simulink model "CraneModel_Final"  (R2022b)
settings: Solver=FixedStepAuto  StartTime=0.0  StopTime=15  FixedStep=0.002  RelTol=1e-3
values from neighbouring files (symbols this model uses):
  fHeightKingActLower = 0.161    [craneParameters.m]
  fHeightKingActUpper = 0.130    (= 0.13)    [craneParameters.m]
  fHeightKingSlew = 0.623    [craneParameters.m]
  fHeightKnuckleActLower = 0.160    (= 0.16)    [craneParameters.m]
  fHeightKnuckleActUpper = 0.182    [craneParameters.m]
  fHeightPlatform = 1.402    [craneParameters.m]
  fHeightPlatformKing = 0.09    [craneParameters.m]
  fHeightSlewTop = 0.711    [craneParameters.m]
  fHeightToSheave1 = 0.060    (= 0.06)    [craneParameters.m]
  fHeightToSheave2 = 0.095    [craneParameters.m]
  fHeightToSheave3 = 0.198    [craneParameters.m]
  fHeightToSheave4 = 1.158    [craneParameters.m]
  fHeightToWinch = 0.0895    [craneParameters.m]
  fLengthKingActLower = 0.154    [craneParameters.m]
  fLengthKingActUpper = 0.600    (= 0.6)    [craneParameters.m]
  fLengthKnuckleActLower = 0.750    (= 0.75)    [craneParameters.m]
  fLengthKnuckleActUpper = 0.027    [craneParameters.m]
  fLengthMainArm = 1.5    [craneParameters.m]
  fLengthPlatform = 1.30    (= 1.3)    [craneParameters.m]
  fLengthToSheave1 = 0.235    [craneParameters.m]
  fLengthToSheave2 = 1.520    (= 1.52)    [craneParameters.m]
  fLengthToSheave3 = 0.168    [craneParameters.m]
  fLengthToSheave4 = 0    [craneParameters.m]
  fLengthToWinch = 0.22    [craneParameters.m]
  fMinLengthActuatorKnuckle = 0.633    [craneParameters.m]
  fMinLengthActuatorMain = 0.691    [craneParameters.m]
  massActuatorBottomMain = 14    [craneParameters.m]
  massActuatorBottomRod = 3    [craneParameters.m]
  massActuatorTopMain = 14    [craneParameters.m]
  massKingBottom = 92.2    [craneParameters.m]
  massKingMountingPlate = 58.2    [craneParameters.m]
  massKingTop = 63.6    [craneParameters.m]
  massKnuckleArm = 8.7    [craneParameters.m]
  massMainArm = 12.5    [craneParameters.m]
  massPayload = 13.5    [craneParameters.m]
  massTestRigBase = 924    [craneParameters.m]
  massTestRigPlatform = 268    [craneParameters.m]
  massWinch = 4.8    [craneParameters.m]
  massWinchDrum = 2.3    [craneParameters.m]
  sheavePitchRadius = sheavePitchDiameter/2    (= 0.034)    [craneParameters.m]
  winchGearRatio = 32    [craneParameters.m]    (also in winchCalculations.m)
undefined symbols (not defined in the file or in its folder): X, Y, Z
libraries: sm_lib x138, nesl_utility x20, vrlib x1, sldrtlib x1
(part 4 of 4)

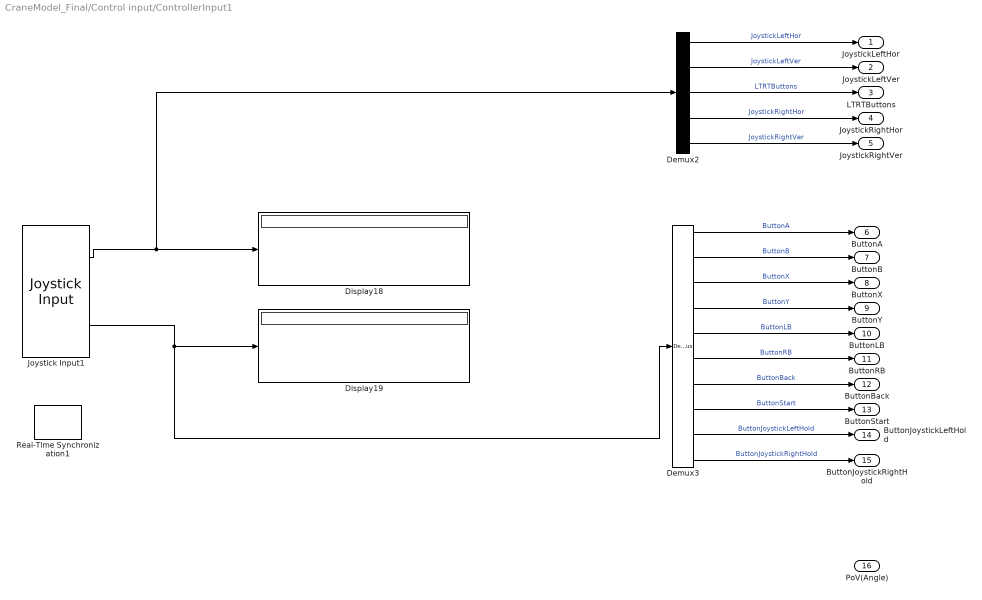
== system CraneModel_Final/Control input/ControllerInput1 ==
  Demux2 : Demux  Outputs=5
  Demux3 : Demux  Outputs=10
  Display18 : Display
  Display19 : Display
  Joystick Input1 : vrlib/Joystick Input  joyid=1  adjustports=on  forcefeed=off
  Real-Time Synchronization1 : sldrtlib/Real-Time Synchronization  SampleTime=0.002  MaxMissedTicks=1000000  ShowMissedTicks=off  YieldWhenWaiting=off
  JoystickLeftHor : Outport
  JoystickLeftVer : Outport  Port=2
  LTRTButtons : Outport  Port=3
  JoystickRightHor : Outport  Port=4
  JoystickRightVer : Outport  Port=5
  ButtonA : Outport  Port=6
  ButtonB : Outport  Port=7
  ButtonX : Outport  Port=8
  ButtonY : Outport  Port=9
  ButtonLB : Outport  Port=10
  ButtonRB : Outport  Port=11
  ButtonBack : Outport  Port=12
  ButtonStart : Outport  Port=13
  ButtonJoystickLeftHold : Outport  Port=14
  ButtonJoystickRightHold : Outport  Port=15
  PoV(Angle) : Outport  Port=16
  wires:
  Joystick Input1/2 -> Display19/1, Demux3/1
  Demux3/1 -> ButtonA/1  "ButtonA"
  Joystick Input1/1 -> Demux2/1, Display18/1
  Demux2/2 -> JoystickLeftVer/1  "JoystickLeftVer"
  Demux2/3 -> LTRTButtons/1  "LTRTButtons"
  Demux3/5 -> ButtonLB/1  "ButtonLB"
  Demux3/3 -> ButtonX/1  "ButtonX"
  Demux2/1 -> JoystickLeftHor/1  "JoystickLeftHor"
  Demux3/10 -> ButtonJoystickRightHold/1  "ButtonJoystickRightHold"
  Demux3/6 -> ButtonRB/1  "ButtonRB"
  Demux2/4 -> JoystickRightHor/1  "JoystickRightHor"
  Demux3/9 -> ButtonJoystickLeftHold/1  "ButtonJoystickLeftHold"
  ? -> PoV(Angle)/1  "PoV(Angle)"
  Demux2/5 -> JoystickRightVer/1  "JoystickRightVer"
  Demux3/7 -> ButtonBack/1  "ButtonBack"
  Demux3/8 -> ButtonStart/1  "ButtonStart"
  Demux3/4 -> ButtonY/1  "ButtonY"
  Demux3/2 -> ButtonB/1  "ButtonB"

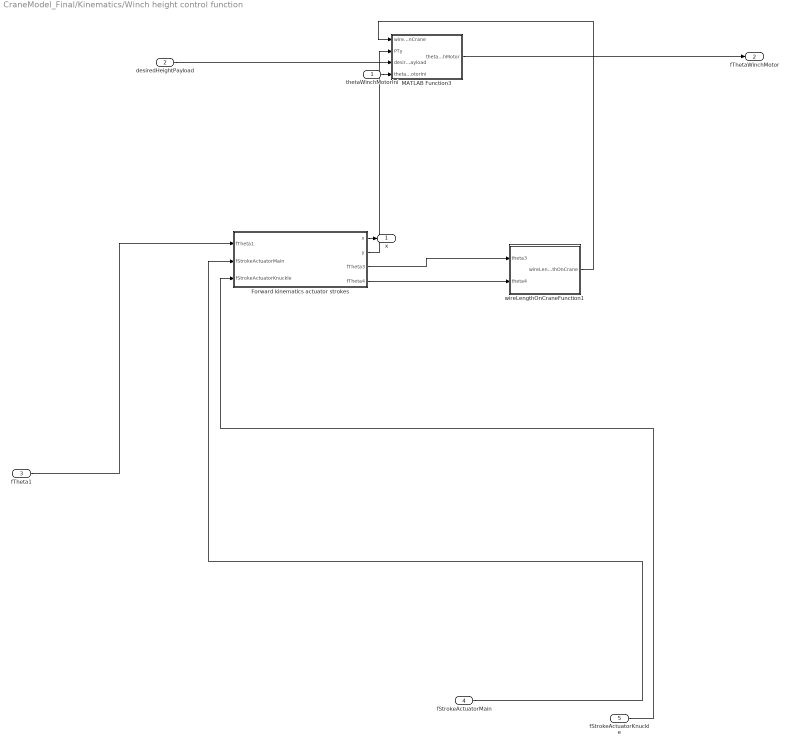
== system CraneModel_Final/Kinematics/Winch height control function ==
  thetaWinchMotorIni : Inport
  desiredHeightPayload : Inport  Port=2
  fTheta1 : Inport  Port=3
  fStrokeActuatorMain : Inport  Port=4
  fStrokeActuatorKnuckle : Inport  Port=5
  Forward kinematics actuator strokes : MATLAB Function  TreatAsAtomicUnit=on
  MATLAB Function3 : MATLAB Function  TreatAsAtomicUnit=on
  wireLengthOnCraneFunction1 : MATLAB Function  TreatAsAtomicUnit=on
  x : Outport
  fThetaWinchMotor : Outport  Port=2
  wires:
  MATLAB Function3/1(thetaWinchMotor) -> fThetaWinchMotor/1
  wireLengthOnCraneFunction1/1(wireLengthOnCrane) -> MATLAB Function3/1(wireLengthOnCrane)
  fStrokeActuatorKnuckle/1 -> Forward kinematics actuator strokes/3(fStrokeActuatorKnuckle)
  Forward kinematics actuator strokes/4(fTheta4) -> wireLengthOnCraneFunction1/2(theta4)
  desiredHeightPayload/1 -> MATLAB Function3/3(desiredHeightPayload)
  fStrokeActuatorMain/1 -> Forward kinematics actuator strokes/2(fStrokeActuatorMain)
  Forward kinematics actuator strokes/2(y) -> MATLAB Function3/2(PTy)
  Forward kinematics actuator strokes/3(fTheta3) -> wireLengthOnCraneFunction1/1(theta3)
  Forward kinematics actuator strokes/1(x) -> x/1
  thetaWinchMotorIni/1 -> MATLAB Function3/4(thetaWinchMotorIni)
  fTheta1/1 -> Forward kinematics actuator strokes/1(fTheta1)

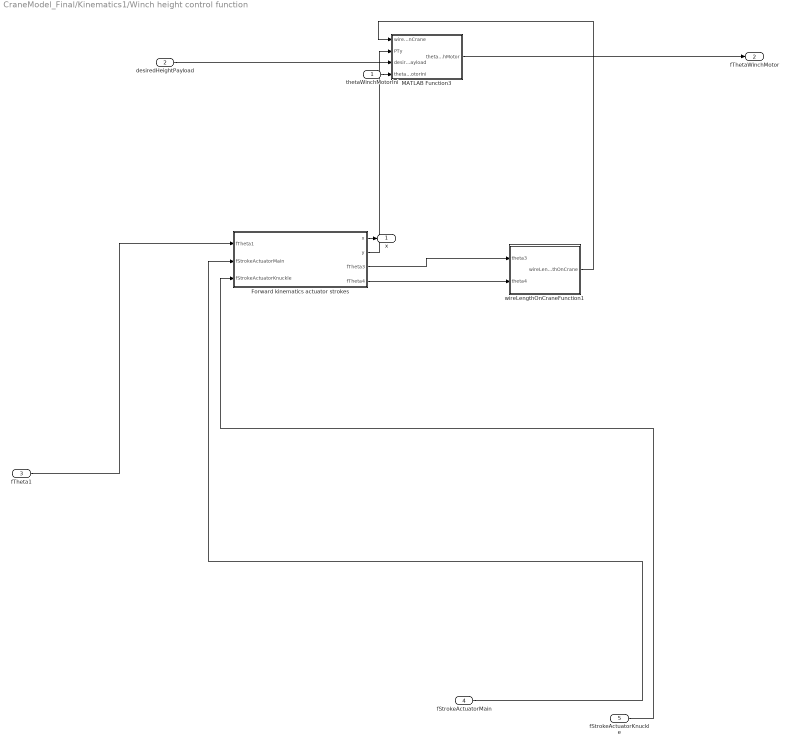
== system CraneModel_Final/Kinematics1/Winch height control function ==
  thetaWinchMotorIni : Inport
  desiredHeightPayload : Inport  Port=2
  fTheta1 : Inport  Port=3
  fStrokeActuatorMain : Inport  Port=4
  fStrokeActuatorKnuckle : Inport  Port=5
  Forward kinematics actuator strokes : MATLAB Function  TreatAsAtomicUnit=on
  MATLAB Function3 : MATLAB Function  TreatAsAtomicUnit=on
  wireLengthOnCraneFunction1 : MATLAB Function  TreatAsAtomicUnit=on
  x : Outport
  fThetaWinchMotor : Outport  Port=2
  wires:
  MATLAB Function3/1(thetaWinchMotor) -> fThetaWinchMotor/1
  wireLengthOnCraneFunction1/1(wireLengthOnCrane) -> MATLAB Function3/1(wireLengthOnCrane)
  fStrokeActuatorKnuckle/1 -> Forward kinematics actuator strokes/3(fStrokeActuatorKnuckle)
  Forward kinematics actuator strokes/4(fTheta4) -> wireLengthOnCraneFunction1/2(theta4)
  desiredHeightPayload/1 -> MATLAB Function3/3(desiredHeightPayload)
  fStrokeActuatorMain/1 -> Forward kinematics actuator strokes/2(fStrokeActuatorMain)
  Forward kinematics actuator strokes/2(y) -> MATLAB Function3/2(PTy)
  Forward kinematics actuator strokes/3(fTheta3) -> wireLengthOnCraneFunction1/1(theta3)
  Forward kinematics actuator strokes/1(x) -> x/1
  thetaWinchMotorIni/1 -> MATLAB Function3/4(thetaWinchMotorIni)
  fTheta1/1 -> Forward kinematics actuator strokes/1(fTheta1)

== matlab function CraneModel_Final/Kinematics/Winch height control function/Forward kinematics actuator strokes ==
  data: fTheta1 input; x output; y output; fStrokeActuatorMain input; fStrokeActuatorKnuckle input; fTheta3 output; fTheta4 output
function [x, y, fTheta3, fTheta4] = fcn(fTheta1, fStrokeActuatorMain, fStrokeActuatorKnuckle)

 %Platform constants
fHeightPlatform = 1.402;
fHeightPlatformKing = 0.09;
fLengthPlatform = 1.30;

%Crane and platform dimensions
%Crane constant parameters

fHeightKingSlew             = 0.623;
fHeightSlewTop              = 0.711;
fLengthMainArm			    = 1.5;
fLengthKnuckleArm		    = 1.158;

fLengthAMain				= 0.614;
fLengthBMain				= 0.571;
fMinLengthActuatorMain		= 0.691;
fMaxStrokeActuatorMain		= 0.320;

fOffsetAngleDegMainAct		= 62.1;
fOffsetAngleRadMainAct		= deg2rad(fOffsetAngleDegMainAct);

fLengthAKnuckle				= 0.767;
fLengthBKnuckle				= 0.184;
fMinLengthActuatorKnuckle	= 0.633;
fMaxStrokeActuatorKnuckle	= 0.260;

fOffsetAngleDegKnuckleAct	= 86.3;
fOffsetAngleRadKnuckleAct	= deg2rad(fOffsetAngleDegKnuckleAct);

%Calculating angles for main arm
fLengthActuatorMain = fStrokeActuatorMain + fMinLengthActuatorMain;

fAngleMainArmAct = acos((fLengthBMain^2 + fLengthAMain^2 - fLengthActuatorMain^2) / (2 * fLengthBMain * fLengthAMain));

fTheta3 = fAngleMainArmAct - fOffsetAngleRadMainAct;

%Calculating angles for knuckle arm
fLengthActuatorKnuckle = fStrokeActuatorKnuckle + fMinLengthActuatorKnuckle;

fAngleKnuckleArmAct = acos((fLengthBKnuckle^2 + fLengthAKnuckle^2 - fLengthActuatorKnuckle^2) / (2 * fLengthBKnuckle * fLengthAKnuckle));

fTheta4 = fAngleKnuckleArmAct - fOffsetAngleRadKnuckleAct;


	
% 
% fAngleMainArmAct			= fTheta3deg + fOffsetAngleDegMainAct;
% fAngleKnuckleArmAct         = fTheta4deg + fOffsetAngleDegKnuckleAct;
% 
% fLengthActuatorMain         = sqrt(fLengthAMain^2 + fLengthBMain^2 -(2*fLengthAMain*fLengthBMain*cosd(fAngleMainArmAct)));
% fStrokeActuatorMain         = fLengthActuatorMain - fMinLengthActuatorMain;
% if fStrokeActuatorMain < 0
%     fStrokeActuatorMain = 0;
% elseif fStrokeActuatorMain > fMaxStrokeActuatorMain
%     fMaxStrokeActuatorMain = fMaxStrokeActuatorMain;
% end
% 
% fLengthActuatorKnuckle         = sqrt(fLengthAKnuckle^2 + fLengthBKnuckle^2 -(2*fLengthAKnuckle*fLengthBKnuckle*cosd(fAngleKnuckleArmAct)));
% fStrokeActuatorKnuckle         = fLengthActuatorKnuckle - fMinLengthActuatorKnuckle;
% 
% if fStrokeActuatorKnuckle < 0
%     fStrokeActuatorKnuckle = 0;
% elseif fStrokeActuatorKnuckle > fMaxStrokeActuatorKnuckle
%     fMaxStrokeActuatorKnuckle = fMaxStrokeActuatorKnuckle;
% end



fHeightMain                 = fHeightPlatformKing + fHeightKingSlew + fHeightSlewTop;

% x = fLengthPlatform*cos(fTheta1) + fHeightMain*cos(fTheta1 + pi/2) + fLengthMainArm*cos(fTheta1 + fTheta3) + fLengthKnuckleArm * cos (fTheta1 + fTheta3 + fTheta4 - pi/2);
% y = fHeightPlatform + fLengthPlatform*sin(fTheta1) + fHeightMain * sin(fTheta1 + pi/2) + fLengthMainArm *sin(fTheta1 + fTheta3) + fLengthKnuckleArm*sin(fTheta1 + fTheta3 + fTheta4 - pi/2);

x = fLengthPlatform*cos(fTheta1) + fHeightMain*cos(fTheta1 + pi/2) + fLengthMainArm*cos(fTheta1 + fTheta3) + fLengthKnuckleArm * cos (fTheta1 + fTheta3 + fTheta4 - pi/2);
y = fHeightPlatform + fLengthPlatform*sin(fTheta1) + fHeightMain * sin(fTheta1 + pi/2) + fLengthMainArm *sin(fTheta1 + fTheta3) + fLengthKnuckleArm*sin(fTheta1 + fTheta3 + fTheta4 - pi/2);

== matlab function CraneModel_Final/Kinematics/WinchHeightControlFunction ==
  data: fTheta1 input; PTx output; PTy output; fStrokeActuatorMain input; fStrokeActuatorKnuckle input; fTheta3 output; fTheta4 output; thetaWinchMotorIni input; desiredHeightPayload input; thetaWinchMotor output
function [PTx, PTy, fTheta3, fTheta4, thetaWinchMotor] = fcn(fTheta1, fStrokeActuatorMain, fStrokeActuatorKnuckle, thetaWinchMotorIni, desiredHeightPayload)

 %Platform constants
fHeightPlatform = 1.402;
fHeightPlatformKing = 0.09;
fLengthPlatform = 1.30;

%Crane and platform dimensions
%Crane constant parameters

fHeightKingSlew             = 0.623;
fHeightSlewTop              = 0.711;
fLengthMainArm			    = 1.5;
fLengthKnuckleArm		    = 1.158;

fLengthAMain				= 0.614;
fLengthBMain				= 0.571;
fMinLengthActuatorMain		= 0.691;
fMaxStrokeActuatorMain		= 0.320;

fOffsetAngleDegMainAct		= 62.1;
fOffsetAngleRadMainAct		= deg2rad(fOffsetAngleDegMainAct);

fLengthAKnuckle				= 0.767;
fLengthBKnuckle				= 0.184;
fMinLengthActuatorKnuckle	= 0.633;
fMaxStrokeActuatorKnuckle	= 0.260;

fOffsetAngleDegKnuckleAct	= 86.3;
fOffsetAngleRadKnuckleAct	= deg2rad(fOffsetAngleDegKnuckleAct);

lengthOrigoToWinch = 0.2199;
heightOrigoToWinch = 0.0895;
lengthOrigoToSheave1 = 0.2348;
heightOrigoToSheave1 = 0.060;
lengthOrigoToSheave2 = 1.520;
heigthOrigoToSheave2 = 0.095;
lengthMainArmToSheave3 = 0.2591;
lengthMainArmToSheave4 = 1.158;
offsetAngleSheave3deg = 49.7;
offsetAngleSheave3rad = deg2rad(offsetAngleSheave3deg);
offsetAngleSheave4deg = 90;
offsetAngleSheave4rad = deg2rad(offsetAngleSheave4deg);

lengthMainArm = 1.500;
pitchRadiusWinch = 0.0716;
pitchRadiusSheave = 0.034;

%Calculating angles for main arm
fLengthActuatorMain = fStrokeActuatorMain + fMinLengthActuatorMain;

fAngleMainArmAct = acos((fLengthBMain^2 + fLengthAMain^2 - fLengthActuatorMain^2) / (2 * fLengthBMain * fLengthAMain));

fTheta3 = fAngleMainArmAct - fOffsetAngleRadMainAct;

%Calculating angles for knuckle arm
fLengthActuatorKnuckle = fStrokeActuatorKnuckle + fMinLengthActuatorKnuckle;

fAngleKnuckleArmAct = acos((fLengthBKnuckle^2 + fLengthAKnuckle^2 - fLengthActuatorKnuckle^2) / (2 * fLengthBKnuckle * fLengthAKnuckle));

fTheta4 = fAngleKnuckleArmAct - fOffsetAngleRadKnuckleAct;


fHeightMain = fHeightPlatformKing + fHeightKingSlew + fHeightSlewTop;

PTx = fLengthPlatform*cos(fTheta1) + fHeightMain*cos(fTheta1 + pi/2) + fLengthMainArm*cos(fTheta1 + fTheta3) + fLengthKnuckleArm * cos (fTheta1 + fTheta3 + fTheta4 - pi/2);
PTy = fHeightPlatform + fLengthPlatform*sin(fTheta1) + fHeightMain * sin(fTheta1 + pi/2) + fLengthMainArm *sin(fTheta1 + fTheta3) + fLengthKnuckleArm*sin(fTheta1 + fTheta3 + fTheta4 - pi/2);


Pwx = -lengthOrigoToWinch;
Pwy = -heightOrigoToWinch;
Ps1x = lengthOrigoToSheave1 * cos(fTheta3) - heightOrigoToSheave1 * sin(fTheta3);
Ps1y = lengthOrigoToSheave1 * sin(fTheta3) + heightOrigoToSheave1 * cos(fTheta3);
Ps2x = lengthOrigoToSheave2 * cos(fTheta3) - heigthOrigoToSheave2 * sin(fTheta3);
Ps2y = lengthOrigoToSheave2 * sin(fTheta3) + heigthOrigoToSheave2 * cos(fTheta3);
Ps3x = lengthMainArm * cos(fTheta3) + lengthMainArmToSheave3 * cos(fTheta3 + fTheta4 - offsetAngleSheave3rad);
Ps3y = lengthMainArm * sin(fTheta3) + lengthMainArmToSheave3 * sin(fTheta3 + fTheta4 - offsetAngleSheave3rad); 
Ps4x = lengthMainArm * cos(fTheta3) + lengthMainArmToSheave4 * cos(fTheta3 + fTheta4 - offsetAngleSheave4rad);
Ps4y = lengthMainArm * sin(fTheta3) + lengthMainArmToSheave4 * sin(fTheta3 + fTheta4 - offsetAngleSheave4rad);

%  function distance = distanceTwoPoints(P1x, P1y, P2x, P2y)
%        distance = sqrt((P2x - P1x)^2 + (P2y - P1y)^2);
%    end

distanceWinchSheave1 =  sqrt((Ps1x - Pwx)^2 + (Ps1y - Pwy)^2); %distanceTwoPoints(Pwx, Pwy, Ps1x, Ps1y);
distanceSheave1Sheave2 = sqrt((Ps2x - Ps1x)^2 + (Ps2y - Ps1y)^2); %distanceTwoPoints(Ps2x, Ps2y, Ps1x, Ps1y);
distanceSheave2Sheave3 = sqrt((Ps3x - Ps2x)^2 + (Ps3y - Ps2y)^2); %distanceTwoPoints(Ps2x, Ps2y, Ps3x, Ps3y);
distanceSheave3Sheave4 = sqrt((Ps4x - Ps3x)^2 + (Ps4y - Ps3y)^2); %distanceTwoPoints(Ps4x, Ps4y, Ps3x, Ps3y);

% function tangentLength = tangentLengthFunction(distance, radius1, radius2)
%         tangentLength = sqrt(distance^2 -(radius1 -radius2)^2);
%     end

tangentLengthWinchSheave1 = sqrt(distanceWinchSheave1^2 -(pitchRadiusWinch -pitchRadiusSheave)^2); %tangentLengthFunction(distanceWinchSheave1, pitchRadiusWinch, pitchRadiusSheave);
tangentLengthSheave1Sheave2 = sqrt(distanceSheave1Sheave2^2 -(pitchRadiusSheave -pitchRadiusSheave)^2); %tangentLengthFunction(distanceSheave1Sheave2, pitchRadiusSheave, pitchRadiusSheave);
tangentLengthSheave2Sheave3 = sqrt(distanceSheave2Sheave3^2 -(pitchRadiusSheave -pitchRadiusSheave)^2); %tangentLengthFunction(distanceSheave2Sheave3, pitchRadiusSheave, pitchRadiusSheave);
tangentLengthSheave3Sheave4 = sqrt(distanceSheave3Sheave4^2 -(pitchRadiusSheave -pitchRadiusSheave)^2); %tangentLengthFunction(distanceSheave3Sheave4, pitchRadiusSheave, pitchRadiusSheave);

offsetAngleDeg = 113.6 + 9.9;
offsetAngleRad = deg2rad(offsetAngleDeg);

wrapAngle = offsetAngleRad - fTheta3 - fTheta4;
wrapLength = wrapAngle * pitchRadiusSheave;

wireLengthOnCrane = tangentLengthWinchSheave1 + tangentLengthSheave1Sheave2 + tangentLengthSheave2Sheave3 + tangentLengthSheave3Sheave4 + wrapLength;

lengthWinchWireIni = 3;
pitchRadiusWinch = 0.0716;
pitchRadiusSheave = 0.034;
gearRatioWinch = 32;

lengthWinchWire = PTy - desiredHeightPayload;
thetaWinch = (lengthWinchWire - lengthWinchWireIni) / pitchRadiusWinch;
thetaWinchMotor = thetaWinch*gearRatioWinch + thetaWinchMotorIni;

%     function distance = distanceTwoPoints(P1x, P1y, P2x, P2y)
%         distance = sqrt((P2x - P1x)^2 + (P2y - P1y)^2);
%     end
% 
%     function tangentLength = tangentLengthFunction(distance, radius1, radius2)
%         tangentLength = sqrt(distance^2 -(radius1 -radius2)^2);
%     end
end

== matlab function CraneModel_Final/Kinematics1/Inverse kinematics function ==
  data: fPtXd input; fPtYd input; fStrokeActuatorMain output; fStrokeActuatorKnuckle output; fTheta1 input; fTheta3 output; fTheta4 output
function [fStrokeActuatorMain, fStrokeActuatorKnuckle, fTheta3, fTheta4] = fcn(fPtXd, fPtYd, fTheta1)
    
    %Platform constants
    h0 = 1.402;
    l0 = 1.3;
    
    %Crane constants
    h1 = 1.334 + 0.09;
    lm = 1.5;
    lk = 1.158;

    %Calculate position of a2 as function of Theta1
    a2x = l0*cos(fTheta1) + h1*cos(fTheta1 + pi/2);
    a2y = h0 + l0*sin(fTheta1) + h1*sin(fTheta1 + pi/2);

    h = sqrt((fPtXd - a2x)^2 + (fPtYd - a2y)^2);
    phi = atan((fPtYd - a2y) / (fPtXd - a2x));
    
    %Calculate ThetaA and ThetaB
    ThetaA = acos ((lm^2 + h^2 - lk^2) / (2*lm*h));
    ThetaB = acos ((lk^2 + lm^2 - h^2) / (2*lm*lk));

    fTheta3 = ThetaA + phi - fTheta1;
    fTheta4 = ThetaB - pi/2;

    fTheta3deg = rad2deg(fTheta3);
    fTheta4deg = rad2deg(fTheta4);

	%Crane constant parameters
	fLengthP2PMainArm			= lm;
	fLengthP2PKnuckleArm		= lk;
	
	fLengthAMain				= 0.614;
	fLengthBMain				= 0.571;
	fMinLengthActuatorMain		= 0.691;
	fMaxStrokeActuatorMain		= 0.320;
	
    fOffsetAngleDegMainAct		= 62.1;
	
	fLengthAKnuckle				= 0.767;
	fLengthBKnuckle				= 0.184;
	fMinLengthActuatorKnuckle	= 0.633;
	fMaxStrokeActuatorKnuckle	= 0.260;
	
    fOffsetAngleDegKnuckleAct	= 86.3;
	

fAngleMainArmAct			= fTheta3deg + fOffsetAngleDegMainAct;
fAngleKnuckleArmAct         = fTheta4deg + fOffsetAngleDegKnuckleAct;

fLengthActuatorMain         = sqrt(fLengthAMain^2 + fLengthBMain^2 -(2*fLengthAMain*fLengthBMain*cosd(fAngleMainArmAct)));
fStrokeActuatorMain         = fLengthActuatorMain - fMinLengthActuatorMain;

if fStrokeActuatorMain < 0
    fStrokeActuatorMain = 0;
elseif fStrokeActuatorMain > fMaxStrokeActuatorMain
    fMaxStrokeActuatorMain = fMaxStrokeActuatorMain;
end

fLengthActuatorKnuckle         = sqrt(fLengthAKnuckle^2 + fLengthBKnuckle^2 -(2*fLengthAKnuckle*fLengthBKnuckle*cosd(fAngleKnuckleArmAct)));
fStrokeActuatorKnuckle         = fLengthActuatorKnuckle - fMinLengthActuatorKnuckle;

if fStrokeActuatorKnuckle < 0
    fStrokeActuatorKnuckle = 0;
elseif fStrokeActuatorKnuckle > fMaxStrokeActuatorKnuckle
    fMaxStrokeActuatorKnuckle = fMaxStrokeActuatorKnuckle;
end

== matlab function CraneModel_Final/Kinematics1/Winch height control function/Forward kinematics actuator strokes ==
  data: fTheta1 input; x output; y output; fStrokeActuatorMain input; fStrokeActuatorKnuckle input; fTheta3 output; fTheta4 output
function [x, y, fTheta3, fTheta4] = fcn(fTheta1, fStrokeActuatorMain, fStrokeActuatorKnuckle)

 %Platform constants
fHeightPlatform = 1.402;
fHeightPlatformKing = 0.09;
fLengthPlatform = 1.30;

%Crane and platform dimensions
%Crane constant parameters

fHeightKingSlew             = 0.623;
fHeightSlewTop              = 0.711;
fLengthMainArm			    = 1.5;
fLengthKnuckleArm		    = 1.158;

fLengthAMain				= 0.614;
fLengthBMain				= 0.571;
fMinLengthActuatorMain		= 0.691;
fMaxStrokeActuatorMain		= 0.320;

fOffsetAngleDegMainAct		= 62.1;
fOffsetAngleRadMainAct		= deg2rad(fOffsetAngleDegMainAct);

fLengthAKnuckle				= 0.767;
fLengthBKnuckle				= 0.184;
fMinLengthActuatorKnuckle	= 0.633;
fMaxStrokeActuatorKnuckle	= 0.260;

fOffsetAngleDegKnuckleAct	= 86.3;
fOffsetAngleRadKnuckleAct	= deg2rad(fOffsetAngleDegKnuckleAct);

%Calculating angles for main arm
fLengthActuatorMain = fStrokeActuatorMain + fMinLengthActuatorMain;

fAngleMainArmAct = acos((fLengthBMain^2 + fLengthAMain^2 - fLengthActuatorMain^2) / (2 * fLengthBMain * fLengthAMain));

fTheta3 = fAngleMainArmAct - fOffsetAngleRadMainAct;

%Calculating angles for knuckle arm
fLengthActuatorKnuckle = fStrokeActuatorKnuckle + fMinLengthActuatorKnuckle;

fAngleKnuckleArmAct = acos((fLengthBKnuckle^2 + fLengthAKnuckle^2 - fLengthActuatorKnuckle^2) / (2 * fLengthBKnuckle * fLengthAKnuckle));

fTheta4 = fAngleKnuckleArmAct - fOffsetAngleRadKnuckleAct;


	
% 
% fAngleMainArmAct			= fTheta3deg + fOffsetAngleDegMainAct;
% fAngleKnuckleArmAct         = fTheta4deg + fOffsetAngleDegKnuckleAct;
% 
% fLengthActuatorMain         = sqrt(fLengthAMain^2 + fLengthBMain^2 -(2*fLengthAMain*fLengthBMain*cosd(fAngleMainArmAct)));
% fStrokeActuatorMain         = fLengthActuatorMain - fMinLengthActuatorMain;
% if fStrokeActuatorMain < 0
%     fStrokeActuatorMain = 0;
% elseif fStrokeActuatorMain > fMaxStrokeActuatorMain
%     fMaxStrokeActuatorMain = fMaxStrokeActuatorMain;
% end
% 
% fLengthActuatorKnuckle         = sqrt(fLengthAKnuckle^2 + fLengthBKnuckle^2 -(2*fLengthAKnuckle*fLengthBKnuckle*cosd(fAngleKnuckleArmAct)));
% fStrokeActuatorKnuckle         = fLengthActuatorKnuckle - fMinLengthActuatorKnuckle;
% 
% if fStrokeActuatorKnuckle < 0
%     fStrokeActuatorKnuckle = 0;
% elseif fStrokeActuatorKnuckle > fMaxStrokeActuatorKnuckle
%     fMaxStrokeActuatorKnuckle = fMaxStrokeActuatorKnuckle;
% end



fHeightMain                 = fHeightPlatformKing + fHeightKingSlew + fHeightSlewTop;

% x = fLengthPlatform*cos(fTheta1) + fHeightMain*cos(fTheta1 + pi/2) + fLengthMainArm*cos(fTheta1 + fTheta3) + fLengthKnuckleArm * cos (fTheta1 + fTheta3 + fTheta4 - pi/2);
% y = fHeightPlatform + fLengthPlatform*sin(fTheta1) + fHeightMain * sin(fTheta1 + pi/2) + fLengthMainArm *sin(fTheta1 + fTheta3) + fLengthKnuckleArm*sin(fTheta1 + fTheta3 + fTheta4 - pi/2);

x = fLengthPlatform*cos(fTheta1) + fHeightMain*cos(fTheta1 + pi/2) + fLengthMainArm*cos(fTheta1 + fTheta3) + fLengthKnuckleArm * cos (fTheta1 + fTheta3 + fTheta4 - pi/2);
y = fHeightPlatform + fLengthPlatform*sin(fTheta1) + fHeightMain * sin(fTheta1 + pi/2) + fLengthMainArm *sin(fTheta1 + fTheta3) + fLengthKnuckleArm*sin(fTheta1 + fTheta3 + fTheta4 - pi/2);

== matlab function CraneModel_Final/Kinematics1/Winch height control function/MATLAB Function3 ==
  data: wireLengthOnCrane input; PTy input; thetaWinchMotor output; desiredHeightPayload input; thetaWinchMotorIni input
function thetaWinchMotor = fcn(wireLengthOnCrane, PTy, desiredHeightPayload, thetaWinchMotorIni)

lengthWinchWireIni = 3;
pitchRadiusWinch = 0.0716;
pitchRadiusSheave = 0.034;
gearRatioWinch = 32;

lengthWinchWire = PTy - desiredHeightPayload;
thetaWinch = (lengthWinchWire - lengthWinchWireIni) / pitchRadiusWinch;
thetaWinchMotor = thetaWinch*gearRatioWinch + thetaWinchMotorIni;

== matlab function CraneModel_Final/Kinematics1/Winch height control function/wireLengthOnCraneFunction1 ==
  data: theta3 input; wireLengthOnCrane output; theta4 input
function wireLengthOnCrane = fcn(theta3, theta4)

lengthOrigoToWinch = 0.2199;
heightOrigoToWinch = 0.0895;
lengthOrigoToSheave1 = 0.2348;
heightOrigoToSheave1 = 0.060;
lengthOrigoToSheave2 = 1.520;
heigthOrigoToSheave2 = 0.095;
lengthMainArmToSheave3 = 0.2591;
lengthMainArmToSheave4 = 1.158;
offsetAngleSheave3deg = 49.7;
offsetAngleSheave3rad = deg2rad(offsetAngleSheave3deg);
offsetAngleSheave4deg = 90;
offsetAngleSheave4rad = deg2rad(offsetAngleSheave4deg);

lengthMainArm = 1.500;
pitchRadiusWinch = 0.0716;
pitchRadiusSheave = 0.034;

Pwx = -lengthOrigoToWinch;
Pwy = -heightOrigoToWinch;
Ps1x = lengthOrigoToSheave1 * cos(theta3) - heightOrigoToSheave1 * sin(theta3);
Ps1y = lengthOrigoToSheave1 * sin(theta3) + heightOrigoToSheave1 * cos(theta3);
Ps2x = lengthOrigoToSheave2 * cos(theta3) - heigthOrigoToSheave2 * sin(theta3);
Ps2y = lengthOrigoToSheave2 * sin(theta3) + heigthOrigoToSheave2 * cos(theta3);
Ps3x = lengthMainArm * cos(theta3) + lengthMainArmToSheave3 * cos(theta3 + theta4 - offsetAngleSheave3rad);
Ps3y = lengthMainArm * sin(theta3) + lengthMainArmToSheave3 * sin(theta3 + theta4 - offsetAngleSheave3rad); 
Ps4x = lengthMainArm * cos(theta3) + lengthMainArmToSheave4 * cos(theta3 + theta4 - offsetAngleSheave4rad);
Ps4y = lengthMainArm * sin(theta3) + lengthMainArmToSheave4 * sin(theta3 + theta4 - offsetAngleSheave4rad);

distanceWinchSheave1 = distanceTwoPoints(Pwx, Pwy, Ps1x, Ps1y);
distanceSheave1Sheave2 = distanceTwoPoints(Ps2x, Ps2y, Ps1x, Ps1y);
distanceSheave2Sheave3 = distanceTwoPoints(Ps2x, Ps2y, Ps3x, Ps3y);
distanceSheave3Sheave4 = distanceTwoPoints(Ps4x, Ps4y, Ps3x, Ps3y);

tangentLengthWinchSheave1 = tangentLengthFunction(distanceWinchSheave1, pitchRadiusWinch, pitchRadiusSheave);
tangentLengthSheave1Sheave2 = tangentLengthFunction(distanceSheave1Sheave2, pitchRadiusSheave, pitchRadiusSheave);
tangentLengthSheave2Sheave3 = tangentLengthFunction(distanceSheave2Sheave3, pitchRadiusSheave, pitchRadiusSheave);
tangentLengthSheave3Sheave4 = tangentLengthFunction(distanceSheave3Sheave4, pitchRadiusSheave, pitchRadiusSheave);

offsetAngleDeg = 113.6 + 9.9;
offsetAngleRad = deg2rad(offsetAngleDeg);

wrapAngle = offsetAngleRad - theta3 - theta4;
wrapLength = wrapAngle * pitchRadiusSheave;

wireLengthOnCrane = tangentLengthWinchSheave1 + tangentLengthSheave1Sheave2 + tangentLengthSheave2Sheave3 + tangentLengthSheave3Sheave4 + wrapLength;

    function distance = distanceTwoPoints(P1x, P1y, P2x, P2y)
        distance = sqrt((P2x - P1x)^2 + (P2y - P1y)^2);
    end

    function tangentLength = tangentLengthFunction(distance, radius1, radius2)
        tangentLength = sqrt(distance^2 -(radius1 -radius2)^2);
    end
end

== matlab function CraneModel_Final/Kinematics1/WinchHeightControlFunction ==
  data: fTheta1 input; PTx output; PTy output; fStrokeActuatorMain input; fStrokeActuatorKnuckle input; fTheta3 output; fTheta4 output; thetaWinchMotorIni input; desiredHeightPayload input; thetaWinchMotor output
function [PTx, PTy, fTheta3, fTheta4, thetaWinchMotor] = fcn(fTheta1, fStrokeActuatorMain, fStrokeActuatorKnuckle, thetaWinchMotorIni, desiredHeightPayload)

 %Platform constants
fHeightPlatform = 1.402;
fHeightPlatformKing = 0.09;
fLengthPlatform = 1.30;

%Crane and platform dimensions
%Crane constant parameters

fHeightKingSlew             = 0.623;
fHeightSlewTop              = 0.711;
fLengthMainArm			    = 1.5;
fLengthKnuckleArm		    = 1.158;

fLengthAMain				= 0.614;
fLengthBMain				= 0.571;
fMinLengthActuatorMain		= 0.691;
fMaxStrokeActuatorMain		= 0.320;

fOffsetAngleDegMainAct		= 62.1;
fOffsetAngleRadMainAct		= deg2rad(fOffsetAngleDegMainAct);

fLengthAKnuckle				= 0.767;
fLengthBKnuckle				= 0.184;
fMinLengthActuatorKnuckle	= 0.633;
fMaxStrokeActuatorKnuckle	= 0.260;

fOffsetAngleDegKnuckleAct	= 86.3;
fOffsetAngleRadKnuckleAct	= deg2rad(fOffsetAngleDegKnuckleAct);

lengthOrigoToWinch = 0.2199;
heightOrigoToWinch = 0.0895;
lengthOrigoToSheave1 = 0.2348;
heightOrigoToSheave1 = 0.060;
lengthOrigoToSheave2 = 1.520;
heigthOrigoToSheave2 = 0.095;
lengthMainArmToSheave3 = 0.2591;
lengthMainArmToSheave4 = 1.158;
offsetAngleSheave3deg = 49.7;
offsetAngleSheave3rad = deg2rad(offsetAngleSheave3deg);
offsetAngleSheave4deg = 90;
offsetAngleSheave4rad = deg2rad(offsetAngleSheave4deg);

lengthMainArm = 1.500;
pitchRadiusWinch = 0.0716;
pitchRadiusSheave = 0.034;

%Calculating angles for main arm
fLengthActuatorMain = fStrokeActuatorMain + fMinLengthActuatorMain;

fAngleMainArmAct = acos((fLengthBMain^2 + fLengthAMain^2 - fLengthActuatorMain^2) / (2 * fLengthBMain * fLengthAMain));

fTheta3 = fAngleMainArmAct - fOffsetAngleRadMainAct;

%Calculating angles for knuckle arm
fLengthActuatorKnuckle = fStrokeActuatorKnuckle + fMinLengthActuatorKnuckle;

fAngleKnuckleArmAct = acos((fLengthBKnuckle^2 + fLengthAKnuckle^2 - fLengthActuatorKnuckle^2) / (2 * fLengthBKnuckle * fLengthAKnuckle));

fTheta4 = fAngleKnuckleArmAct - fOffsetAngleRadKnuckleAct;


fHeightMain = fHeightPlatformKing + fHeightKingSlew + fHeightSlewTop;

PTx = fLengthPlatform*cos(fTheta1) + fHeightMain*cos(fTheta1 + pi/2) + fLengthMainArm*cos(fTheta1 + fTheta3) + fLengthKnuckleArm * cos (fTheta1 + fTheta3 + fTheta4 - pi/2);
PTy = fHeightPlatform + fLengthPlatform*sin(fTheta1) + fHeightMain * sin(fTheta1 + pi/2) + fLengthMainArm *sin(fTheta1 + fTheta3) + fLengthKnuckleArm*sin(fTheta1 + fTheta3 + fTheta4 - pi/2);


Pwx = -lengthOrigoToWinch;
Pwy = -heightOrigoToWinch;
Ps1x = lengthOrigoToSheave1 * cos(fTheta3) - heightOrigoToSheave1 * sin(fTheta3);
Ps1y = lengthOrigoToSheave1 * sin(fTheta3) + heightOrigoToSheave1 * cos(fTheta3);
Ps2x = lengthOrigoToSheave2 * cos(fTheta3) - heigthOrigoToSheave2 * sin(fTheta3);
Ps2y = lengthOrigoToSheave2 * sin(fTheta3) + heigthOrigoToSheave2 * cos(fTheta3);
Ps3x = lengthMainArm * cos(fTheta3) + lengthMainArmToSheave3 * cos(fTheta3 + fTheta4 - offsetAngleSheave3rad);
Ps3y = lengthMainArm * sin(fTheta3) + lengthMainArmToSheave3 * sin(fTheta3 + fTheta4 - offsetAngleSheave3rad); 
Ps4x = lengthMainArm * cos(fTheta3) + lengthMainArmToSheave4 * cos(fTheta3 + fTheta4 - offsetAngleSheave4rad);
Ps4y = lengthMainArm * sin(fTheta3) + lengthMainArmToSheave4 * sin(fTheta3 + fTheta4 - offsetAngleSheave4rad);

%  function distance = distanceTwoPoints(P1x, P1y, P2x, P2y)
%        distance = sqrt((P2x - P1x)^2 + (P2y - P1y)^2);
%    end

distanceWinchSheave1 =  sqrt((Ps1x - Pwx)^2 + (Ps1y - Pwy)^2); %distanceTwoPoints(Pwx, Pwy, Ps1x, Ps1y);
distanceSheave1Sheave2 = sqrt((Ps2x - Ps1x)^2 + (Ps2y - Ps1y)^2); %distanceTwoPoints(Ps2x, Ps2y, Ps1x, Ps1y);
distanceSheave2Sheave3 = sqrt((Ps3x - Ps2x)^2 + (Ps3y - Ps2y)^2); %distanceTwoPoints(Ps2x, Ps2y, Ps3x, Ps3y);
distanceSheave3Sheave4 = sqrt((Ps4x - Ps3x)^2 + (Ps4y - Ps3y)^2); %distanceTwoPoints(Ps4x, Ps4y, Ps3x, Ps3y);

% function tangentLength = tangentLengthFunction(distance, radius1, radius2)
%         tangentLength = sqrt(distance^2 -(radius1 -radius2)^2);
%     end

tangentLengthWinchSheave1 = sqrt(distanceWinchSheave1^2 -(pitchRadiusWinch -pitchRadiusSheave)^2); %tangentLengthFunction(distanceWinchSheave1, pitchRadiusWinch, pitchRadiusSheave);
tangentLengthSheave1Sheave2 = sqrt(distanceSheave1Sheave2^2 -(pitchRadiusSheave -pitchRadiusSheave)^2); %tangentLengthFunction(distanceSheave1Sheave2, pitchRadiusSheave, pitchRadiusSheave);
tangentLengthSheave2Sheave3 = sqrt(distanceSheave2Sheave3^2 -(pitchRadiusSheave -pitchRadiusSheave)^2); %tangentLengthFunction(distanceSheave2Sheave3, pitchRadiusSheave, pitchRadiusSheave);
tangentLengthSheave3Sheave4 = sqrt(distanceSheave3Sheave4^2 -(pitchRadiusSheave -pitchRadiusSheave)^2); %tangentLengthFunction(distanceSheave3Sheave4, pitchRadiusSheave, pitchRadiusSheave);

offsetAngleDeg = 113.6 + 9.9;
offsetAngleRad = deg2rad(offsetAngleDeg);

wrapAngle = offsetAngleRad - fTheta3 - fTheta4;
wrapLength = wrapAngle * pitchRadiusSheave;

wireLengthOnCrane = tangentLengthWinchSheave1 + tangentLengthSheave1Sheave2 + tangentLengthSheave2Sheave3 + tangentLengthSheave3Sheave4 + wrapLength;

lengthWinchWireIni = 3;
pitchRadiusWinch = 0.0716;
pitchRadiusSheave = 0.034;
gearRatioWinch = 32;

lengthWinchWire = PTy - desiredHeightPayload;
thetaWinch = (lengthWinchWire - lengthWinchWireIni) / pitchRadiusWinch;
thetaWinchMotor = thetaWinch*gearRatioWinch + thetaWinchMotorIni;

%     function distance = distanceTwoPoints(P1x, P1y, P2x, P2y)
%         distance = sqrt((P2x - P1x)^2 + (P2y - P1y)^2);
%     end
% 
%     function tangentLength = tangentLengthFunction(distance, radius1, radius2)
%         tangentLength = sqrt(distance^2 -(radius1 -radius2)^2);
%     end
end

== matlab function CraneModel_Final/Kinematics/Winch height control function/MATLAB Function3 ==
  data: wireLengthOnCrane input; PTy input; thetaWinchMotor output; desiredHeightPayload input; thetaWinchMotorIni input
function thetaWinchMotor = fcn(wireLengthOnCrane, PTy, desiredHeightPayload, thetaWinchMotorIni)

lengthWinchWireIni = 3;
pitchRadiusWinch = 0.0716;
pitchRadiusSheave = 0.034;
gearRatioWinch = 32;

lengthWinchWire = PTy - desiredHeightPayload;
thetaWinch = (lengthWinchWire - lengthWinchWireIni) / pitchRadiusWinch;
thetaWinchMotor = thetaWinch*gearRatioWinch + thetaWinchMotorIni;

== matlab function CraneModel_Final/Kinematics/Inverse kinematics function ==
  data: fPtXd input; fPtYd input; fStrokeActuatorMain output; fStrokeActuatorKnuckle output; fTheta1 input; fTheta3 output; fTheta4 output
function [fStrokeActuatorMain, fStrokeActuatorKnuckle, fTheta3, fTheta4] = fcn(fPtXd, fPtYd, fTheta1)

   
    %Platform constants
    h0 = 1.402;
    l0 = 1.3;
    
    %Crane constants
    h1 = 1.334 + 0.09;
    lm = 1.5;
    lk = 1.158;

    %Calculate position of a2 as function of Theta1
    a2x = l0*cos(fTheta1) + h1*cos(fTheta1 + pi/2);
    a2y = h0 + l0*sin(fTheta1) + h1*sin(fTheta1 + pi/2);

    h = sqrt((fPtXd - a2x)^2 + (fPtYd - a2y)^2);
    phi = atan((fPtYd - a2y) / (fPtXd - a2x));
    
    %Calculate ThetaA and ThetaB
    ThetaA = acos ((lm^2 + h^2 - lk^2) / (2*lm*h));
    ThetaB = acos ((lk^2 + lm^2 - h^2) / (2*lm*lk));

    fTheta3 = ThetaA + phi - fTheta1;
    fTheta4 = ThetaB - pi/2;

    fTheta3deg = rad2deg(fTheta3);
    fTheta4deg = rad2deg(fTheta4);

	%Crane constant parameters
	fLengthP2PMainArm			= lm;
	fLengthP2PKnuckleArm		= lk;
	
	fLengthAMain				= 0.614;
	fLengthBMain				= 0.571;
	fMinLengthActuatorMain		= 0.691;
	fMaxStrokeActuatorMain		= 0.320;
	
    fOffsetAngleDegMainAct		= 62.1;
	
	fLengthAKnuckle				= 0.767;
	fLengthBKnuckle				= 0.184;
	fMinLengthActuatorKnuckle	= 0.633;
	fMaxStrokeActuatorKnuckle	= 0.260;
	
    fOffsetAngleDegKnuckleAct	= 86.3;
	

fAngleMainArmAct			= fTheta3deg + fOffsetAngleDegMainAct;
fAngleKnuckleArmAct         = fTheta4deg + fOffsetAngleDegKnuckleAct;

fLengthActuatorMain         = sqrt(fLengthAMain^2 + fLengthBMain^2 -(2*fLengthAMain*fLengthBMain*cosd(fAngleMainArmAct)));
fStrokeActuatorMain         = fLengthActuatorMain - fMinLengthActuatorMain;

if fStrokeActuatorMain < 0
    fStrokeActuatorMain = 0;
elseif fStrokeActuatorMain > fMaxStrokeActuatorMain
    fMaxStrokeActuatorMain = fMaxStrokeActuatorMain;
end

fLengthActuatorKnuckle         = sqrt(fLengthAKnuckle^2 + fLengthBKnuckle^2 -(2*fLengthAKnuckle*fLengthBKnuckle*cosd(fAngleKnuckleArmAct)));
fStrokeActuatorKnuckle         = fLengthActuatorKnuckle - fMinLengthActuatorKnuckle;

if fStrokeActuatorKnuckle < 0
    fStrokeActuatorKnuckle = 0;
elseif fStrokeActuatorKnuckle > fMaxStrokeActuatorKnuckle
    fMaxStrokeActuatorKnuckle = fMaxStrokeActuatorKnuckle;
end

== matlab function CraneModel_Final/Kinematics/Winch height control function/wireLengthOnCraneFunction1 ==
  data: theta3 input; wireLengthOnCrane output; theta4 input
function wireLengthOnCrane = fcn(theta3, theta4)

lengthOrigoToWinch = 0.2199;
heightOrigoToWinch = 0.0895;
lengthOrigoToSheave1 = 0.2348;
heightOrigoToSheave1 = 0.060;
lengthOrigoToSheave2 = 1.520;
heigthOrigoToSheave2 = 0.095;
lengthMainArmToSheave3 = 0.2591;
lengthMainArmToSheave4 = 1.158;
offsetAngleSheave3deg = 49.7;
offsetAngleSheave3rad = deg2rad(offsetAngleSheave3deg);
offsetAngleSheave4deg = 90;
offsetAngleSheave4rad = deg2rad(offsetAngleSheave4deg);

lengthMainArm = 1.500;
pitchRadiusWinch = 0.0716;
pitchRadiusSheave = 0.034;

Pwx = -lengthOrigoToWinch;
Pwy = -heightOrigoToWinch;
Ps1x = lengthOrigoToSheave1 * cos(theta3) - heightOrigoToSheave1 * sin(theta3);
Ps1y = lengthOrigoToSheave1 * sin(theta3) + heightOrigoToSheave1 * cos(theta3);
Ps2x = lengthOrigoToSheave2 * cos(theta3) - heigthOrigoToSheave2 * sin(theta3);
Ps2y = lengthOrigoToSheave2 * sin(theta3) + heigthOrigoToSheave2 * cos(theta3);
Ps3x = lengthMainArm * cos(theta3) + lengthMainArmToSheave3 * cos(theta3 + theta4 - offsetAngleSheave3rad);
Ps3y = lengthMainArm * sin(theta3) + lengthMainArmToSheave3 * sin(theta3 + theta4 - offsetAngleSheave3rad); 
Ps4x = lengthMainArm * cos(theta3) + lengthMainArmToSheave4 * cos(theta3 + theta4 - offsetAngleSheave4rad);
Ps4y = lengthMainArm * sin(theta3) + lengthMainArmToSheave4 * sin(theta3 + theta4 - offsetAngleSheave4rad);

distanceWinchSheave1 = distanceTwoPoints(Pwx, Pwy, Ps1x, Ps1y);
distanceSheave1Sheave2 = distanceTwoPoints(Ps2x, Ps2y, Ps1x, Ps1y);
distanceSheave2Sheave3 = distanceTwoPoints(Ps2x, Ps2y, Ps3x, Ps3y);
distanceSheave3Sheave4 = distanceTwoPoints(Ps4x, Ps4y, Ps3x, Ps3y);

tangentLengthWinchSheave1 = tangentLengthFunction(distanceWinchSheave1, pitchRadiusWinch, pitchRadiusSheave);
tangentLengthSheave1Sheave2 = tangentLengthFunction(distanceSheave1Sheave2, pitchRadiusSheave, pitchRadiusSheave);
tangentLengthSheave2Sheave3 = tangentLengthFunction(distanceSheave2Sheave3, pitchRadiusSheave, pitchRadiusSheave);
tangentLengthSheave3Sheave4 = tangentLengthFunction(distanceSheave3Sheave4, pitchRadiusSheave, pitchRadiusSheave);

offsetAngleDeg = 113.6 + 9.9;
offsetAngleRad = deg2rad(offsetAngleDeg);

wrapAngle = offsetAngleRad - theta3 - theta4;
wrapLength = wrapAngle * pitchRadiusSheave;

wireLengthOnCrane = tangentLengthWinchSheave1 + tangentLengthSheave1Sheave2 + tangentLengthSheave2Sheave3 + tangentLengthSheave3Sheave4 + wrapLength;

    function distance = distanceTwoPoints(P1x, P1y, P2x, P2y)
        distance = sqrt((P2x - P1x)^2 + (P2y - P1y)^2);
    end

    function tangentLength = tangentLengthFunction(distance, radius1, radius2)
        tangentLength = sqrt(distance^2 -(radius1 -radius2)^2);
    end
end
